simulink model "furuta_sim_L"  (R2020b)
settings: Solver=VariableStepAuto  StartTime=0.0  StopTime=5  MaxStep=1e-3  RelTol=1e-3
values from neighbouring files (symbols this model uses):
  A = A1    [furuta_script.m]    (also in practica2.m = [0 1; -2 -3])
  B = B1    [furuta_script.m]    (also in practica2.m = [10; 20])
  b1 = 1.00e-4    (= 0.0001)    [parameters.m]
  b2 = 2.80e-4    (= 0.00028)    [parameters.m]
  C = [1 0 0 0 0; 0 1 0 0 0]    [parameters.m]    (also in practica2.m = [1 0])
  CI = [-5*pi/180 -pi*5/180 0 0 0]    [furuta_script.m]
  g = 9.81    [parameters.m]
  J_hat_0 = J_hat_1+m2*L1^2    (= 0.0373463)    [parameters.m]
  J_hat_2 = J2+m2*l2^2    (= 0.0055028)    [parameters.m]
  Km = 0.090    (= 0.09)    [parameters.m]
  L = 0.005    [parameters.m]    (also in practica2_2.m = acker(Pss.A', Pss.c', Pdl)'; test_delete.m = acker(A',C',po)')
  L1 = 0.278    [parameters.m]
  l2 = 0.148    [parameters.m]
  m2 = 0.075    [parameters.m]
  n = length(A1)    [parameters.m]
  p = width(B1)    [parameters.m]    (also in test_delete.m = roots(conv([1 2*z*wn wn^2], [ 1 alpha*wn])))
  R = 7.80    (= 7.8)    [parameters.m]
undefined symbols (not defined in the file or in its folder): CIL, Lb, Li, Lo
settings Model: Creator=jorgegonzales  LastModifiedBy=jorgegonzales

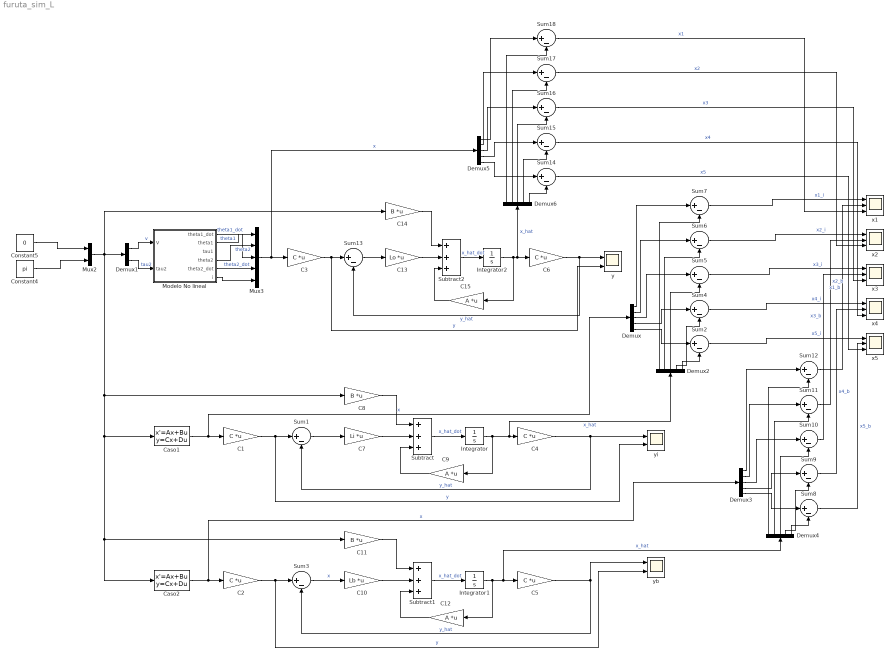
== system furuta_sim_L ==
  C{1..6} (6 alike) : Gain  Gain=C  Multiplication=Matrix(K*u) (u vector)
  C10 : Gain  Gain=Lb  Multiplication=Matrix(K*u) (u vector)
  C11 : Gain  Gain=B  Multiplication=Matrix(K*u) (u vector)
  C12 : Gain  Gain=A  Multiplication=Matrix(K*u) (u vector)
  C13 : Gain  Gain=Lo  Multiplication=Matrix(K*u) (u vector)
  C14 : Gain  Gain=B  Multiplication=Matrix(K*u) (u vector)
  C15 : Gain  Gain=A  Multiplication=Matrix(K*u) (u vector)
  C7 : Gain  Gain=Li  Multiplication=Matrix(K*u) (u vector)
  C8 : Gain  Gain=B  Multiplication=Matrix(K*u) (u vector)
  C9 : Gain  Gain=A  Multiplication=Matrix(K*u) (u vector)
  Caso1 : StateSpace  A=A  B=B  C=eye(n)  D=zeros(n,p)  InitialCondition=CI
  Caso2 : StateSpace  A=A  B=B  C=eye(n)  D=zeros(n,p)  InitialCondition=CI
  Constant4 : Constant  Value=pi
  Constant5 : Constant  Value=0
  Demux{,2..6} (6 alike) : Demux  Outputs=5
  Demux1 : Demux  Outputs=2
  Integrator : Integrator  InitialCondition=CIL
  Integrator1 : Integrator  InitialCondition=CIL
  Integrator2 : Integrator  InitialCondition=CIL
  Modelo No lineal : Subsystem
  Mux2 : Mux  Inputs=2
  Mux3 : Mux  Inputs=5
  Subtract : Sum  Inputs=+++
  Subtract1 : Sum  Inputs=+++
  Subtract2 : Sum  Inputs=+++
  Sum{1..18} (18 alike) : Sum  Inputs=|+-
  x{1..5} (5 alike) : Scope  NumInputPorts=3
  y : Scope  NumInputPorts=2
  yb : Scope  NumInputPorts=2
  yi : Scope  NumInputPorts=2
  wires:
  Caso1/1 -> Demux/1, C1/1  "x"
  Modelo No lineal/2(theta1) -> Mux3/1  "theta1"
  Modelo No lineal/4(theta2) -> Mux3/2  "theta2"
  Modelo No lineal/1(theta1_dot) -> Mux3/3  "theta1_dot"
  Modelo No lineal/5(theta2_dot) -> Mux3/4  "theta2_dot"
  Modelo No lineal/6(i) -> Mux3/5
  Mux3/1 -> Demux5/1, C3/1  "x"
  C4/1 -> yi/1, Sum1/2  "y_hat"
  Constant5/1 -> Mux2/1
  Constant4/1 -> Mux2/2
  Demux1/1 -> Modelo No lineal/1(V)  "v"
  Demux1/2 -> Modelo No lineal/2(tau2)  "tau2"
  Integrator/1 -> C9/1, Demux2/1, C4/1  "x_hat"
  Sum1/1 -> C7/1
  C7/1 -> Subtract/2
  C8/1 -> Subtract/1
  C9/1 -> Subtract/3
  Subtract/1 -> Integrator/1  "x_hat_dot"
  C1/1 -> yi/2, Sum1/1  "y"
  Sum2/1 -> x5/1  "x5_i"
  Demux/5 -> Sum2/1
  Demux2/5 -> Sum2/2
  C2/1 -> yb/2, Sum3/1  "y"
  Subtract1/1 -> Integrator1/1  "x_hat_dot"
  C12/1 -> Subtract1/3
  C11/1 -> Subtract1/1
  C10/1 -> Subtract1/2
  Mux2/1 -> C14/1, Demux1/1, C11/1, Caso2/1, Caso1/1, C8/1
  C5/1 -> Sum3/2, yb/1  "y_hat"
  Caso2/1 -> Demux3/1, C2/1  "x"
  Demux2/4 -> Sum4/2
  Sum4/1 -> x4/1  "x4_i"
  Demux/4 -> Sum4/1
  Demux2/3 -> Sum5/2
  Sum5/1 -> x3/1  "x3_i"
  Demux2/2 -> Sum6/2
  Demux2/1 -> Sum7/2
  Demux/3 -> Sum5/1
  Demux/2 -> Sum6/1
  Demux/1 -> Sum7/1
  Sum7/1 -> x1/1  "x1_i"
  Sum6/1 -> x2/1  "x2_i"
  Sum11/1 -> x2/2  "x2_b"
  Sum12/1 -> x1/2  "x1_b"
  Demux3/1 -> Sum12/1
  Demux3/2 -> Sum11/1
  Demux3/3 -> Sum10/1
  Demux4/1 -> Sum12/2
  Demux4/2 -> Sum11/2
  Sum10/1 -> x3/2  "x3_b"
  Demux4/3 -> Sum10/2
  Demux3/4 -> Sum9/1
  Sum9/1 -> x4/2  "x4_b"
  Demux4/4 -> Sum9/2
  Demux4/5 -> Sum8/2
  Demux3/5 -> Sum8/1
  Sum8/1 -> x5/2  "x5_b"
  Integrator1/1 -> C5/1, Demux4/1, C12/1  "x_hat"
  Sum3/1 -> C10/1  "x"
  C3/1 -> y/2, Sum13/1  "y"
  Sum13/1 -> C13/1
  C13/1 -> Subtract2/2
  C14/1 -> Subtract2/1
  Subtract2/1 -> Integrator2/1  "x_hat_dot"
  Integrator2/1 -> Demux6/1, C6/1, C15/1  "x_hat"
  C15/1 -> Subtract2/3
  C6/1 -> Sum13/2, y/1  "y_hat"
  Demux6/5 -> Sum14/2
  Demux6/4 -> Sum15/2
  Demux6/3 -> Sum16/2
  Demux6/2 -> Sum17/2
  Demux6/1 -> Sum18/2
  Demux5/5 -> Sum14/1
  Demux5/4 -> Sum15/1
  Demux5/3 -> Sum16/1
  Demux5/2 -> Sum17/1
  Demux5/1 -> Sum18/1
  Sum14/1 -> x5/3  "x5"
  Sum15/1 -> x4/3  "x4"
  Sum16/1 -> x3/3  "x3"
  Sum17/1 -> x2/3  "x2"
  Sum18/1 -> x1/3  "x1"

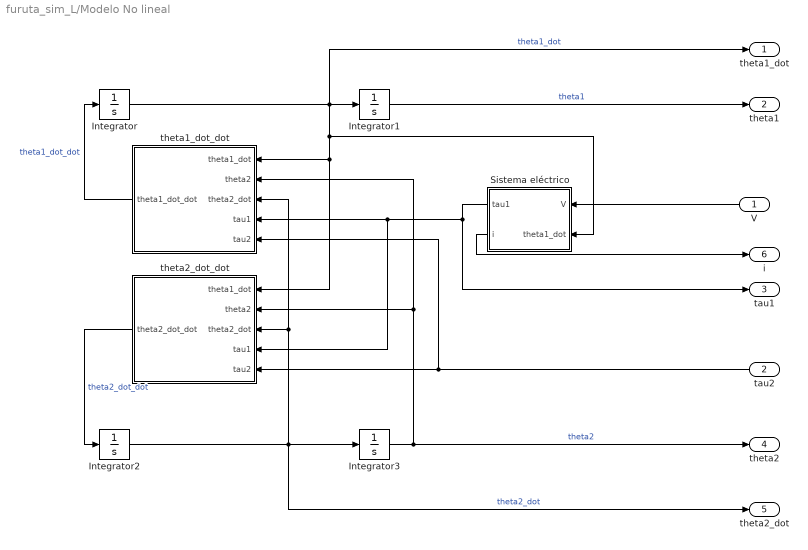
== system furuta_sim_L/Modelo No lineal ==
  V : Inport
  tau2 : Inport  Port=2
  Integrator : Integrator  InitialCondition=CI(3)
  Integrator1 : Integrator  InitialCondition=CI(1)
  Integrator2 : Integrator  InitialCondition=CI(4)
  Integrator3 : Integrator  InitialCondition=CI(2)
  Sistema eléctrico : Subsystem
  theta1_dot_dot : Subsystem
  theta2_dot_dot : Subsystem
  theta1_dot : Outport
  theta1 : Outport  Port=2
  tau1 : Outport  Port=3
  theta2 : Outport  Port=4
  theta2_dot : Outport  Port=5
  i : Outport  Port=6
  wires:
  Sistema eléctrico/1(tau1) -> tau1/1, theta2_dot_dot/4(tau1), theta1_dot_dot/4(tau1)
  theta1_dot_dot/1(theta1_dot_dot) -> Integrator/1  "theta1_dot_dot"
  V/1 -> Sistema eléctrico/1(V)
  Integrator3/1 -> theta2/1, theta2_dot_dot/2(theta2), theta1_dot_dot/2(theta2)  "theta2"
  tau2/1 -> theta1_dot_dot/5(tau2), theta2_dot_dot/5(tau2)
  theta2_dot_dot/1(theta2_dot_dot) -> Integrator2/1  "theta2_dot_dot"
  Integrator1/1 -> theta1/1  "theta1"
  Integrator2/1 -> theta2_dot/1, theta2_dot_dot/3(theta2_dot), theta1_dot_dot/3(theta2_dot), Integrator3/1  "theta2_dot"
  Integrator/1 -> theta1_dot/1, Sistema eléctrico/2(theta1_dot), theta1_dot_dot/1(theta1_dot), theta2_dot_dot/1(theta1_dot), Integrator1/1  "theta1_dot"
  Sistema eléctrico/2(i) -> i/1

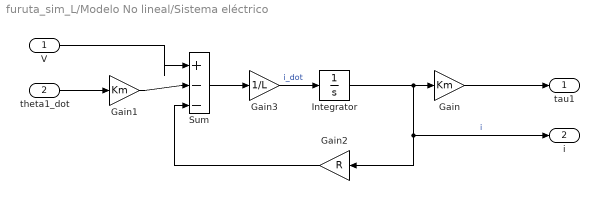
== system furuta_sim_L/Modelo No lineal/Sistema eléctrico ==
  V : Inport
  theta1_dot : Inport  Port=2
  Gain : Gain  Gain=Km
  Gain1 : Gain  Gain=Km
  Gain2 : Gain  Gain=R
  Gain3 : Gain  Gain=1/L
  Integrator : Integrator  InitialCondition=CI(5)
  Sum : Sum  Inputs=|+--
  tau1 : Outport
  i : Outport  Port=2
  wires:
  Integrator/1 -> i/1, Gain2/1, Gain/1  "i"
  Gain/1 -> tau1/1
  theta1_dot/1 -> Gain1/1
  Gain1/1 -> Sum/2
  V/1 -> Sum/1
  Gain2/1 -> Sum/3
  Gain3/1 -> Integrator/1  "i_dot"
  Sum/1 -> Gain3/1

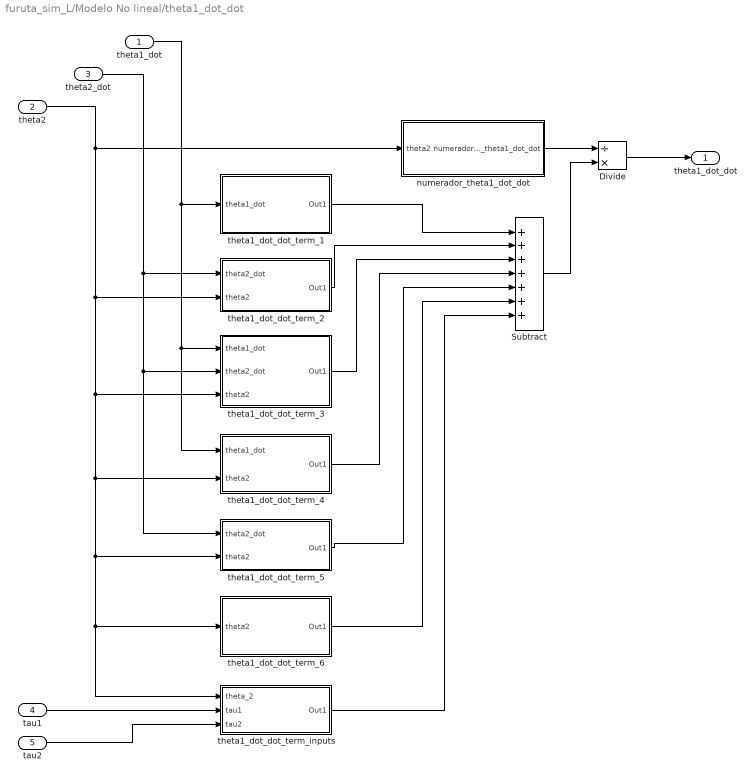
== system furuta_sim_L/Modelo No lineal/theta1_dot_dot ==
  theta1_dot : Inport
  theta2 : Inport  Port=2
  theta2_dot : Inport  Port=3
  tau1 : Inport  Port=4
  tau2 : Inport  Port=5
  Divide : Product  Inputs=/*
  Subtract : Sum  Inputs=+++++++
  numerador_theta1_dot_dot : Subsystem
  theta1_dot_dot_term_1 : Subsystem
  theta1_dot_dot_term_2 : Subsystem
  theta1_dot_dot_term_3 : Subsystem
  theta1_dot_dot_term_4 : Subsystem
  theta1_dot_dot_term_5 : Subsystem
  theta1_dot_dot_term_6 : Subsystem
  theta1_dot_dot_term_inputs : Subsystem
  theta1_dot_dot : Outport
  wires:
  theta1_dot_dot_term_4/1(Out1) -> Subtract/4
  theta1_dot/1 -> theta1_dot_dot_term_3/1(theta1_dot), theta1_dot_dot_term_4/1(theta1_dot), theta1_dot_dot_term_1/1(theta1_dot)
  theta1_dot_dot_term_3/1(Out1) -> Subtract/3
  theta1_dot_dot_term_5/1(Out1) -> Subtract/5
  theta1_dot_dot_term_2/1(Out1) -> Subtract/2
  theta1_dot_dot_term_1/1(Out1) -> Subtract/1
  theta2_dot/1 -> theta1_dot_dot_term_5/1(theta2_dot), theta1_dot_dot_term_3/2(theta2_dot), theta1_dot_dot_term_2/1(theta2_dot)
  theta2/1 -> numerador_theta1_dot_dot/1(theta2), theta1_dot_dot_term_4/2(theta2), theta1_dot_dot_term_6/1(theta2), theta1_dot_dot_term_inputs/1(theta_2), theta1_dot_dot_term_5/2(theta2), theta1_dot_dot_term_3/3(theta2), theta1_dot_dot_term_2/2(theta2)
  tau1/1 -> theta1_dot_dot_term_inputs/2(tau1)
  tau2/1 -> theta1_dot_dot_term_inputs/3(tau2)
  theta1_dot_dot_term_6/1(Out1) -> Subtract/6
  theta1_dot_dot_term_inputs/1(Out1) -> Subtract/7
  numerador_theta1_dot_dot/1(numerador_theta1_dot_dot) -> Divide/1
  Subtract/1 -> Divide/2
  Divide/1 -> theta1_dot_dot/1

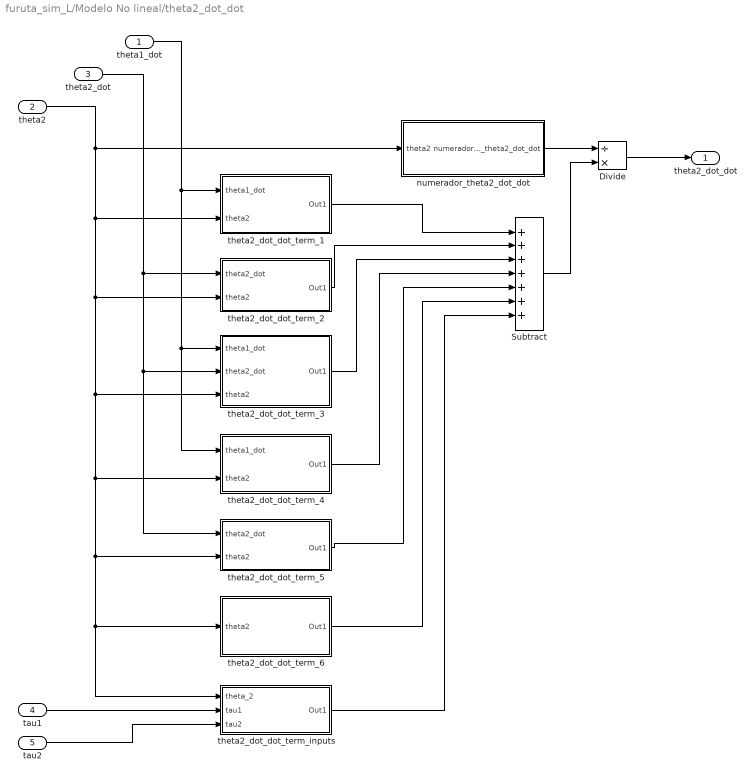
== system furuta_sim_L/Modelo No lineal/theta2_dot_dot ==
  theta1_dot : Inport
  theta2 : Inport  Port=2
  theta2_dot : Inport  Port=3
  tau1 : Inport  Port=4
  tau2 : Inport  Port=5
  Divide : Product  Inputs=/*
  Subtract : Sum  Inputs=+++++++
  numerador_theta2_dot_dot : Subsystem
  theta2_dot_dot_term_1 : Subsystem
  theta2_dot_dot_term_2 : Subsystem
  theta2_dot_dot_term_3 : Subsystem
  theta2_dot_dot_term_4 : Subsystem
  theta2_dot_dot_term_5 : Subsystem
  theta2_dot_dot_term_6 : Subsystem
  theta2_dot_dot_term_inputs : Subsystem
  theta2_dot_dot : Outport
  wires:
  Divide/1 -> theta2_dot_dot/1
  Subtract/1 -> Divide/2
  numerador_theta2_dot_dot/1(numerador_theta2_dot_dot) -> Divide/1
  theta2_dot_dot_term_inputs/1(Out1) -> Subtract/7
  theta2_dot_dot_term_6/1(Out1) -> Subtract/6
  tau2/1 -> theta2_dot_dot_term_inputs/3(tau2)
  tau1/1 -> theta2_dot_dot_term_inputs/2(tau1)
  theta2/1 -> theta2_dot_dot_term_1/2(theta2), theta2_dot_dot_term_2/2(theta2), theta2_dot_dot_term_3/3(theta2), theta2_dot_dot_term_5/2(theta2), theta2_dot_dot_term_inputs/1(theta_2), theta2_dot_dot_term_6/1(theta2), theta2_dot_dot_term_4/2(theta2), numerador_theta2_dot_dot/1(theta2)
  theta2_dot/1 -> theta2_dot_dot_term_2/1(theta2_dot), theta2_dot_dot_term_3/2(theta2_dot), theta2_dot_dot_term_5/1(theta2_dot)
  theta2_dot_dot_term_1/1(Out1) -> Subtract/1
  theta2_dot_dot_term_2/1(Out1) -> Subtract/2
  theta2_dot_dot_term_5/1(Out1) -> Subtract/5
  theta2_dot_dot_term_3/1(Out1) -> Subtract/3
  theta1_dot/1 -> theta2_dot_dot_term_4/1(theta1_dot), theta2_dot_dot_term_3/1(theta1_dot), theta2_dot_dot_term_1/1(theta1_dot)
  theta2_dot_dot_term_4/1(Out1) -> Subtract/4

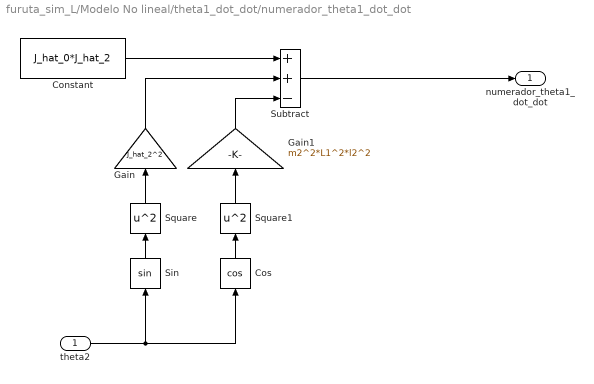
== system furuta_sim_L/Modelo No lineal/theta1_dot_dot/numerador_theta1_dot_dot ==
  theta2 : Inport
  Constant : Constant  Value=J_hat_0*J_hat_2
  Cos : Trigonometry  Operator=cos
  Gain : Gain  Gain=J_hat_2^2
  Gain1 : Gain  Gain=m2^2*L1^2*l2^2
  Sin : Trigonometry
  Square : Math  Operator=square  SaturateOnIntegerOverflow=on
  Square1 : Math  Operator=square  SaturateOnIntegerOverflow=on
  Subtract : Sum  Inputs=++-
  numerador_theta1_dot_dot : Outport
  wires:
  Subtract/1 -> numerador_theta1_dot_dot/1
  Gain1/1 -> Subtract/3
  Sin/1 -> Square/1
  Gain/1 -> Subtract/2
  Constant/1 -> Subtract/1
  theta2/1 -> Cos/1, Sin/1
  Cos/1 -> Square1/1
  Square/1 -> Gain/1
  Square1/1 -> Gain1/1

== system furuta_sim_L/Modelo No lineal/theta1_dot_dot/theta1_dot_dot_term_1 ==
  theta1_dot : Inport
  Gain2 : Gain  Gain=-1*J_hat_2*b1
  Out1 : Outport
  wires:
  theta1_dot/1 -> Gain2/1
  Gain2/1 -> Out1/1

== system furuta_sim_L/Modelo No lineal/theta1_dot_dot/theta1_dot_dot_term_2 ==
  theta2_dot : Inport
  theta2 : Inport  Port=2
  Cos1 : Trigonometry  Operator=cos
  Divide1 : Product  Inputs=**
  Gain3 : Gain  Gain=m2*L1*l2*b2
  Out1 : Outport
  wires:
  Gain3/1 -> Divide1/1
  theta2_dot/1 -> Divide1/2
  Cos1/1 -> Gain3/1
  theta2/1 -> Cos1/1
  Divide1/1 -> Out1/1

== system furuta_sim_L/Modelo No lineal/theta1_dot_dot/theta1_dot_dot_term_3 ==
  theta1_dot : Inport
  theta2_dot : Inport  Port=2
  theta2 : Inport  Port=3
  Divide2 : Product  Inputs=***
  Gain4 : Gain  Gain=2
  Gain5 : Gain  Gain=-1*J_hat_2^2
  Sin1 : Trigonometry
  Out1 : Outport
  wires:
  theta2_dot/1 -> Divide2/3
  Sin1/1 -> Gain5/1
  theta1_dot/1 -> Divide2/2
  Divide2/1 -> Out1/1
  theta2/1 -> Gain4/1
  Gain4/1 -> Sin1/1
  Gain5/1 -> Divide2/1

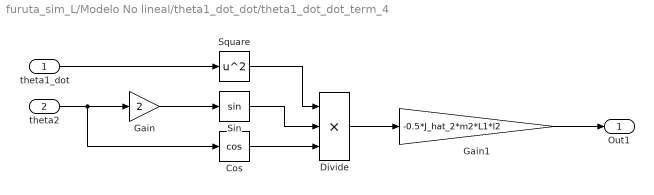
== system furuta_sim_L/Modelo No lineal/theta1_dot_dot/theta1_dot_dot_term_4 ==
  theta1_dot : Inport
  theta2 : Inport  Port=2
  Cos : Trigonometry  Operator=cos
  Divide : Product  Inputs=***
  Gain : Gain  Gain=2
  Gain1 : Gain  Gain=-0.5*J_hat_2*m2*L1*l2
  Sin : Trigonometry
  Square : Math  Operator=square  SaturateOnIntegerOverflow=on
  Out1 : Outport
  wires:
  Gain/1 -> Sin/1
  Divide/1 -> Gain1/1
  theta1_dot/1 -> Square/1
  Square/1 -> Divide/1
  Sin/1 -> Divide/2
  theta2/1 -> Cos/1, Gain/1
  Cos/1 -> Divide/3
  Gain1/1 -> Out1/1

== system furuta_sim_L/Modelo No lineal/theta1_dot_dot/theta1_dot_dot_term_5 ==
  theta2_dot : Inport
  theta2 : Inport  Port=2
  Divide : Product  Inputs=**
  Gain : Gain  Gain=J_hat_2*m2*L1*l2
  Sin : Trigonometry
  Square : Math  Operator=square  SaturateOnIntegerOverflow=on
  Out1 : Outport
  wires:
  theta2_dot/1 -> Square/1
  Square/1 -> Divide/2
  Sin/1 -> Divide/1
  Divide/1 -> Gain/1
  theta2/1 -> Sin/1
  Gain/1 -> Out1/1

== system furuta_sim_L/Modelo No lineal/theta1_dot_dot/theta1_dot_dot_term_6 ==
  theta2 : Inport
  Gain : Gain  Gain=2
  Gain1 : Gain  Gain=0.5*m2^2*l2^2*L1*g
  Sin : Trigonometry
  Out1 : Outport
  wires:
  theta2/1 -> Gain/1
  Gain1/1 -> Out1/1
  Gain/1 -> Sin/1
  Sin/1 -> Gain1/1

== system furuta_sim_L/Modelo No lineal/theta1_dot_dot/theta1_dot_dot_term_inputs ==
  theta_2 : Inport
  tau1 : Inport  Port=2
  tau2 : Inport  Port=3
  Cos : Trigonometry  Operator=cos
  Divide : Product  Inputs=**
  Gain : Gain  Gain=J_hat_2
  Gain1 : Gain  Gain=-1*m2*L1*l2
  Sum : Sum  Inputs=|++
  Out1 : Outport
  wires:
  theta_2/1 -> Cos/1
  Sum/1 -> Out1/1
  Gain/1 -> Sum/1
  Cos/1 -> Divide/2
  tau1/1 -> Gain/1
  tau2/1 -> Divide/1
  Gain1/1 -> Sum/2
  Divide/1 -> Gain1/1

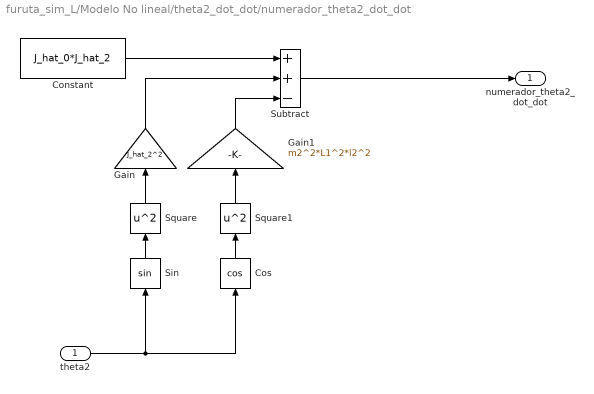
== system furuta_sim_L/Modelo No lineal/theta2_dot_dot/numerador_theta2_dot_dot ==
  theta2 : Inport
  Constant : Constant  Value=J_hat_0*J_hat_2
  Cos : Trigonometry  Operator=cos
  Gain : Gain  Gain=J_hat_2^2
  Gain1 : Gain  Gain=m2^2*L1^2*l2^2
  Sin : Trigonometry
  Square : Math  Operator=square  SaturateOnIntegerOverflow=on
  Square1 : Math  Operator=square  SaturateOnIntegerOverflow=on
  Subtract : Sum  Inputs=++-
  numerador_theta2_dot_dot : Outport
  wires:
  Square1/1 -> Gain1/1
  Square/1 -> Gain/1
  Cos/1 -> Square1/1
  theta2/1 -> Cos/1, Sin/1
  Constant/1 -> Subtract/1
  Gain/1 -> Subtract/2
  Sin/1 -> Square/1
  Gain1/1 -> Subtract/3
  Subtract/1 -> numerador_theta2_dot_dot/1

== system furuta_sim_L/Modelo No lineal/theta2_dot_dot/theta2_dot_dot_term_1 ==
  theta1_dot : Inport
  theta2 : Inport  Port=2
  Cos : Trigonometry  Operator=cos
  Divide : Product  Inputs=**
  Gain2 : Gain  Gain=m2*L1*l2*b1
  Out1 : Outport
  wires:
  Gain2/1 -> Out1/1
  theta2/1 -> Cos/1
  Cos/1 -> Divide/2
  theta1_dot/1 -> Divide/1
  Divide/1 -> Gain2/1

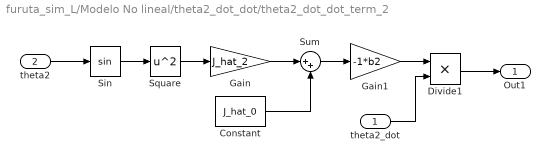
== system furuta_sim_L/Modelo No lineal/theta2_dot_dot/theta2_dot_dot_term_2 ==
  theta2_dot : Inport
  theta2 : Inport  Port=2
  Constant : Constant  Value=J_hat_0
  Divide1 : Product  Inputs=**
  Gain : Gain  Gain=J_hat_2
  Gain1 : Gain  Gain=-1*b2
  Sin : Trigonometry
  Square : Math  Operator=square  SaturateOnIntegerOverflow=on
  Sum : Sum  Inputs=|++
  Out1 : Outport
  wires:
  Divide1/1 -> Out1/1
  theta2/1 -> Sin/1
  Sin/1 -> Square/1
  Square/1 -> Gain/1
  Gain/1 -> Sum/1
  Constant/1 -> Sum/2
  Sum/1 -> Gain1/1
  Gain1/1 -> Divide1/1
  theta2_dot/1 -> Divide1/2

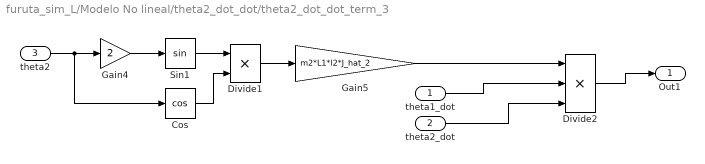
== system furuta_sim_L/Modelo No lineal/theta2_dot_dot/theta2_dot_dot_term_3 ==
  theta1_dot : Inport
  theta2_dot : Inport  Port=2
  theta2 : Inport  Port=3
  Cos : Trigonometry  Operator=cos
  Divide1 : Product  Inputs=**
  Divide2 : Product  Inputs=***
  Gain4 : Gain  Gain=2
  Gain5 : Gain  Gain=m2*L1*l2*J_hat_2
  Sin1 : Trigonometry
  Out1 : Outport
  wires:
  Gain5/1 -> Divide2/1
  Gain4/1 -> Sin1/1
  theta2/1 -> Cos/1, Gain4/1
  Divide2/1 -> Out1/1
  theta1_dot/1 -> Divide2/2
  theta2_dot/1 -> Divide2/3
  Sin1/1 -> Divide1/1
  Cos/1 -> Divide1/2
  Divide1/1 -> Gain5/1

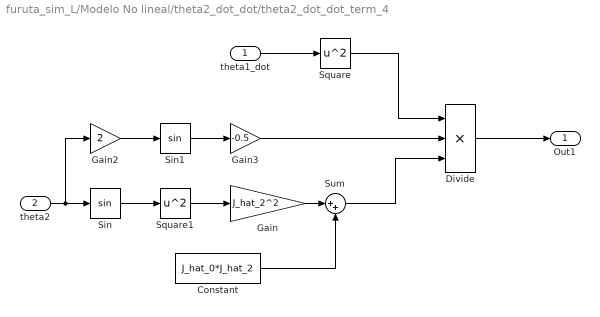
== system furuta_sim_L/Modelo No lineal/theta2_dot_dot/theta2_dot_dot_term_4 ==
  theta1_dot : Inport
  theta2 : Inport  Port=2
  Constant : Constant  Value=J_hat_0*J_hat_2
  Divide : Product  Inputs=***
  Gain : Gain  Gain=J_hat_2^2
  Gain2 : Gain  Gain=2
  Gain3 : Gain  Gain=-0.5
  Sin : Trigonometry
  Sin1 : Trigonometry
  Square : Math  Operator=square  SaturateOnIntegerOverflow=on
  Square1 : Math  Operator=square  SaturateOnIntegerOverflow=on
  Sum : Sum  Inputs=|++
  Out1 : Outport
  wires:
  Divide/1 -> Out1/1
  Square/1 -> Divide/1
  theta1_dot/1 -> Square/1
  theta2/1 -> Gain2/1, Sin/1
  Sin/1 -> Square1/1
  Square1/1 -> Gain/1
  Gain/1 -> Sum/1
  Constant/1 -> Sum/2
  Gain2/1 -> Sin1/1
  Sin1/1 -> Gain3/1
  Gain3/1 -> Divide/2
  Sum/1 -> Divide/3

== system furuta_sim_L/Modelo No lineal/theta2_dot_dot/theta2_dot_dot_term_5 ==
  theta2_dot : Inport
  theta2 : Inport  Port=2
  Divide : Product  Inputs=**
  Gain : Gain  Gain=-0.5*m2^2*L1^2*l2^2
  Gain1 : Gain  Gain=2
  Sin : Trigonometry
  Square : Math  Operator=square  SaturateOnIntegerOverflow=on
  Out1 : Outport
  wires:
  Gain/1 -> Out1/1
  Divide/1 -> Gain/1
  Sin/1 -> Divide/1
  Square/1 -> Divide/2
  theta2_dot/1 -> Square/1
  theta2/1 -> Gain1/1
  Gain1/1 -> Sin/1

== system furuta_sim_L/Modelo No lineal/theta2_dot_dot/theta2_dot_dot_term_6 ==
  theta2 : Inport
  Constant : Constant  Value=J_hat_0
  Divide : Product  Inputs=**
  Gain : Gain  Gain=J_hat_2
  Gain1 : Gain  Gain=-1*m2*l2*g
  Sin : Trigonometry
  Square : Math  Operator=square  SaturateOnIntegerOverflow=on
  Sum : Sum  Inputs=|++
  Out1 : Outport
  wires:
  Gain1/1 -> Out1/1
  theta2/1 -> Sin/1
  Sin/1 -> Divide/1, Square/1
  Square/1 -> Gain/1
  Gain/1 -> Sum/1
  Constant/1 -> Sum/2
  Sum/1 -> Divide/2
  Divide/1 -> Gain1/1

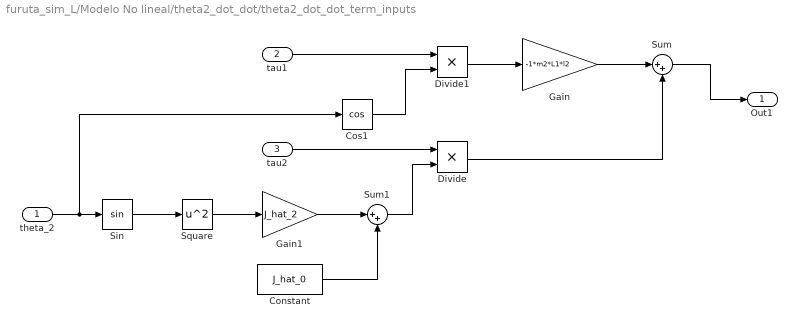
== system furuta_sim_L/Modelo No lineal/theta2_dot_dot/theta2_dot_dot_term_inputs ==
  theta_2 : Inport
  tau1 : Inport  Port=2
  tau2 : Inport  Port=3
  Constant : Constant  Value=J_hat_0
  Cos1 : Trigonometry  Operator=cos
  Divide : Product  Inputs=**
  Divide1 : Product  Inputs=**
  Gain : Gain  Gain=-1*m2*L1*l2
  Gain1 : Gain  Gain=J_hat_2
  Sin : Trigonometry
  Square : Math  Operator=square  SaturateOnIntegerOverflow=on
  Sum : Sum  Inputs=|++
  Sum1 : Sum  Inputs=|++
  Out1 : Outport
  wires:
  Divide/1 -> Sum/2
  tau2/1 -> Divide/1
  Sum/1 -> Out1/1
  tau1/1 -> Divide1/1
  Cos1/1 -> Divide1/2
  Gain/1 -> Sum/1
  Divide1/1 -> Gain/1
  theta_2/1 -> Cos1/1, Sin/1
  Sin/1 -> Square/1
  Square/1 -> Gain1/1
  Gain1/1 -> Sum1/1
  Constant/1 -> Sum1/2
  Sum1/1 -> Divide/2
